simulink model "circuit_electric_RF_model"  (R2025a)
settings: Solver=ode1be  StartTime=0.0  StopTime=Tfin  FixedStep=Ts  RelTol=1e-3
values from neighbouring files (symbols this model uses):
  K = 1.02    [circuit_electric_RF_setup.m]
  t1 = 10    [circuit_electric_RF_setup.m]
  Tfin = 13e-3    (= 0.013)    [circuit_electric_RF_setup.m]
  Ts = 1e-5    (= 1e-05)    [circuit_electric_RF_setup.m]
  u0 = 0    [circuit_electric_RF_setup.m]
  umax = 12    [circuit_electric_RF_setup.m]
  umin = -12    [circuit_electric_RF_setup.m]
  ust = 1    [circuit_electric_RF_setup.m]
  whtn_pow_in = 1e-8/8    (= 1.25e-09)    [circuit_electric_RF_setup.m]
  whtn_pow_out = 1e-8/8    (= 1.25e-09)    [circuit_electric_RF_setup.m]
  whtn_seed_in = 23341    [circuit_electric_RF_setup.m]
  whtn_seed_out = 23342    [circuit_electric_RF_setup.m]
  whtn_Ts_in = Ts    (= 1e-05)    [circuit_electric_RF_setup.m]
  whtn_Ts_out = Ts    (= 1e-05)    [circuit_electric_RF_setup.m]
  wn = 3.1416e+04    (= 31416)    [circuit_electric_RF_setup.m]
  x0 = [1.05,-1000]    [circuit_electric_RF_setup.m]
  ymax = 12    [circuit_electric_RF_setup.m]
  ymin = -12    [circuit_electric_RF_setup.m]
  zeta = 0.35    [circuit_electric_RF_setup.m]
libraries: simulink x5
settings Model: Creator=mircea  LastModifiedBy=mircea

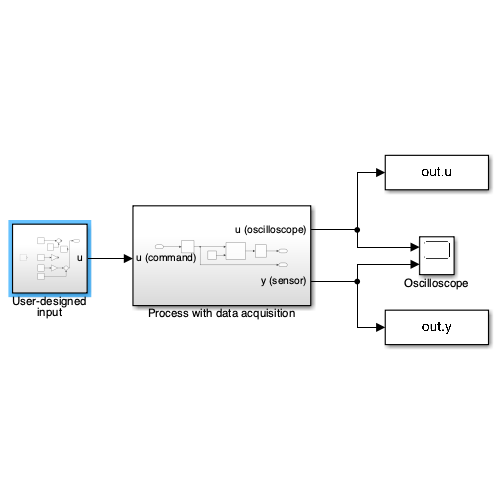
[thumbnail: Simulink's stored preview of the top-level diagram]
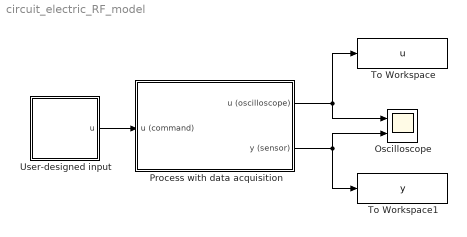
== system circuit_electric_RF_model ==
  Oscilloscope : Scope  NumInputPorts=2
      settings: ActiveDisplayYMinimum=0.74615478515625  ActiveDisplayYMaximum=3.24554443359375
  Process with data acquisition : Subsystem
  To Workspace : ToWorkspace  VariableName=u  SampleTime=Ts
  To Workspace1 : ToWorkspace  VariableName=y  SampleTime=Ts
  User-designed input : Subsystem
  wires:
  Process with data acquisition/1(u (oscilloscope)) -> Oscilloscope/1, To Workspace/1
  Process with data acquisition/2(y (sensor)) -> Oscilloscope/2, To Workspace1/1
  User-designed input/1(u) -> Process with data acquisition/1(u (command))

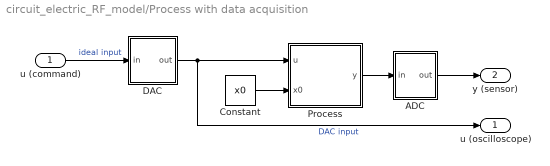
== system circuit_electric_RF_model/Process with data acquisition ==
  u (command) : Inport
  ADC : Subsystem
  Constant : Constant  Value=x0
  DAC : Subsystem
  Process : Subsystem
  u (oscilloscope) : Outport
  y (sensor) : Outport  Port=2
  wires:
  Constant/1 -> Process/2(x0)
  u (command)/1 -> DAC/1(in)  "ideal input"
  Process/1(y) -> ADC/1(in)
  ADC/1(out) -> y (sensor)/1
  DAC/1(out) -> Process/1(u), u (oscilloscope)/1  "DAC input"

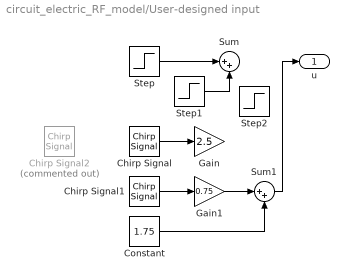
== system circuit_electric_RF_model/User-designed input ==
  Chirp Signal : simulink/Sources/Chirp Signal  f1=0.01  T=80  f2=15
  Chirp Signal1 : simulink/Sources/Chirp Signal  f1=1e2  T=Tfin*1.1  f2=1.0000e+04
  Chirp Signal2 : simulink/Sources/Chirp Signal  Commented=on  f1=1.9231e+03  T=1e-2  f2=1.0000e+04
  Constant : Constant  Value=1.75
  Gain : Gain  Gain=2.5
  Gain1 : Gain  Gain=0.75
  Step : Step  Time=5  Before=u0  After=ust  SampleTime=0
  Step1 : Step  Time=t1  Before=u0  After=ust  SampleTime=0
  Step2 : Step  Time=0  SampleTime=0
  Sum : Sum  Inputs=|++
  Sum1 : Sum  Inputs=|++
  u : Outport
  wires:
  Chirp Signal/1 -> Gain/1
  Step/1 -> Sum/1
  Step1/1 -> Sum/2
  Chirp Signal1/1 -> Gain1/1
  Gain1/1 -> Sum1/1
  Constant/1 -> Sum1/2
  Sum1/1 -> u/1

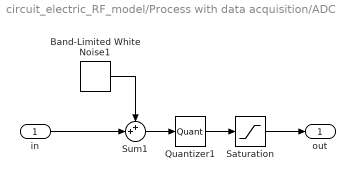
== system circuit_electric_RF_model/Process with data acquisition/ADC ==
  in : Inport
  Band-Limited White Noise1 : simulink/Sources/Band-Limited White Noise  Cov=[whtn_pow_out]  Ts=whtn_Ts_out  seed=[whtn_seed_out]
  Quantizer1 : Quantizer  QuantizationInterval=q_out
  Saturation : Saturate  UpperLimit=ymax  LowerLimit=ymin
  Sum1 : Sum  Inputs=++|
  out : Outport
  wires:
  Quantizer1/1 -> Saturation/1
  Sum1/1 -> Quantizer1/1
  in/1 -> Sum1/2
  Band-Limited White Noise1/1 -> Sum1/1
  Saturation/1 -> out/1

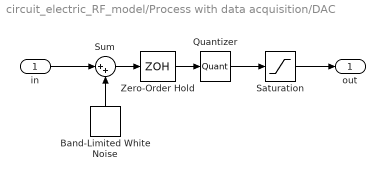
== system circuit_electric_RF_model/Process with data acquisition/DAC ==
  in : Inport
  Band-Limited White Noise : simulink/Sources/Band-Limited White Noise  Cov=[whtn_pow_in]  Ts=whtn_Ts_in  seed=[whtn_seed_in]
  Quantizer : Quantizer  QuantizationInterval=q_in
  Saturation : Saturate  UpperLimit=umax  LowerLimit=umin
  Sum : Sum  Inputs=|++
  Zero-Order Hold : ZeroOrderHold  SampleTime=-1
  out : Outport
  wires:
  Quantizer/1 -> Saturation/1
  Sum/1 -> Zero-Order Hold/1
  in/1 -> Sum/1
  Band-Limited White Noise/1 -> Sum/2
  Zero-Order Hold/1 -> Quantizer/1
  Saturation/1 -> out/1

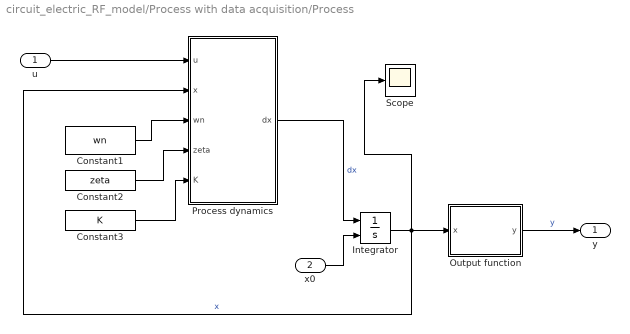
== system circuit_electric_RF_model/Process with data acquisition/Process ==
  u : Inport
  x0 : Inport  Port=2
  Constant1 : Constant  Value=wn
  Constant2 : Constant  Value=zeta
  Constant3 : Constant  Value=K
  Integrator : Integrator  InitialConditionSource=external
  Output function : MATLAB Function  TreatAsAtomicUnit=on
  Process dynamics : MATLAB Function  TreatAsAtomicUnit=on
  Scope : Scope
      settings: ActiveDisplayYMinimum=-30864.820368316767  ActiveDisplayYMaximum=30756.992827113063
  y : Outport
  wires:
  u/1 -> Process dynamics/1(u)
  Process dynamics/1(dx) -> Integrator/1  "dx"
  Integrator/1 -> Scope/1, Output function/1(x), Process dynamics/2(x)  "x"
  Output function/1(y) -> y/1  "y"
  x0/1 -> Integrator/2
  Constant2/1 -> Process dynamics/4(zeta)
  Constant1/1 -> Process dynamics/3(wn)
  Constant3/1 -> Process dynamics/5(K)

== matlab function circuit_electric_RF_model/Process with data acquisition/Process/Process dynamics ==
  data: u input; dx output; x input; wn input; zeta input; K input
function dx = fcn(u,x,wn,zeta,K)
dx = [0,1;
    -wn^2,-2*zeta*wn]*x + [0;K*wn^2]*u;
end

== matlab function circuit_electric_RF_model/Process with data acquisition/Process/Output function ==
  data: y output; x input
function y = fcn(x)

y = x(1);

end
